simulink model "HVAC"  (R2020b)
settings: Solver=VariableStepAuto  StartTime=0.0  StopTime=10.0  RelTol=1e-3
settings Model: PacingRate=0.350000  Creator=Training  LastModifiedBy=Training

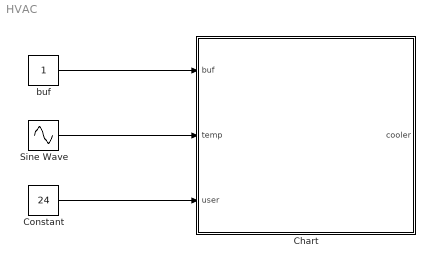
== system HVAC ==
  Chart : Stateflow chart  TreatAsAtomicUnit=on
  Constant : Constant  Value=24
  Sine Wave : Sin  Amplitude=50  SampleTime=0
  buf : Constant
  wires:
  buf/1 -> Chart/1(buf)
  Sine Wave/1 -> Chart/2(temp)
  Constant/1 -> Chart/3(user)

== stateflow chart HVAC/Chart ==
  state NoOperation
    entry:
    power == 1;
  state HeaterOn
    entry:
    heater = 1;
    state ON
      entry:
      state = 1;
    state OFF
      entry:
      state = 0;
    (default) -> ON
    OFF -> ON : [temp-buf<user]{pow=0}
    ON -> OFF : [temp-buf > user]
  state CoolerOn
    entry:
    cooler = 1;
    state ON_C
      entry:
      state_c=1;
    state OFF_C
      entry:
      state_c=0;
    (default) -> ON_C
    OFF_C -> ON_C : [temp+buf >user]{pow= 0}
    ON_C -> OFF_C : [temp+buf < user]
  (default) -> NoOperation
  NoOperation -> HeaterOn [order 1] : [power == 1 && temp-buf<user]
  HeaterOn -> NoOperation : [pow ==0]{power=1}
  CoolerOn -> NoOperation : [pow == 0]
  NoOperation -> CoolerOn [order 2] : [power ==1 && temp+buf>user]
  data: buf input; temp input; user input; cooler output; heater local; state local; state_c local; power local =1; pow local =1
